simulink model "verify_Room_Floor_Heating_mdl"  (R2016b)
settings: Solver=ode15s  StartTime=0  StopTime=24*3600  MaxStep=900  RelTol=1e-3  EnableMultiTasking=on
libraries: carnot x8
settings Model: Creator=drhf  LastModifiedBy=drhf
settings DataIOCC: SaveFormat=Array  SignalLoggingSaveFormat=ModelDataLogs
settings OptimizationCC: ExpressionDepthLimit=2147483647  LifeSpan=inf
settings DebuggingCC: UnderspecifiedInitializationDetection=Classic  MergeDetectMultiDrivingBlocksExec=none  SolverPrmCheckMsg=warning  FcnCallInpInsideContextMsg=warning  StateNameClashWarn=warning  SFUnexpectedBacktrackingDiag=warning  SFNoUnconditionalDefaultTransitionDiag=warning  SFExecutionAtInitializationDiag=none
settings HardwareCC: ProdBitPerPointer=32  ProdBitPerSizeT=32  ProdBitPerPtrDiffT=32  ProdLargestAtomicFloat=None  ProdIntDivRoundTo=Undefined  ProdEndianess=Unspecified  ProdWordSize=32  ProdHWDeviceType=32-bit Generic
settings ModelReferenceCC: PropagateSignalLabelsOutOfModel=off
settings GRTTargetCC: TargetLangStandard=C89/C90 (ANSI)  GeneratePreprocessorConditionals=Disable all  CombineOutputUpdateFcns=off  GRTInterface=on
settings ConfigComp: CovMetricSettings=dw  CovHtmlReporting=on  CovSaveCumulativeToWorkspaceVar=on  CovSaveSingleToWorkspaceVar=on  CovExternalEMLEnable=off

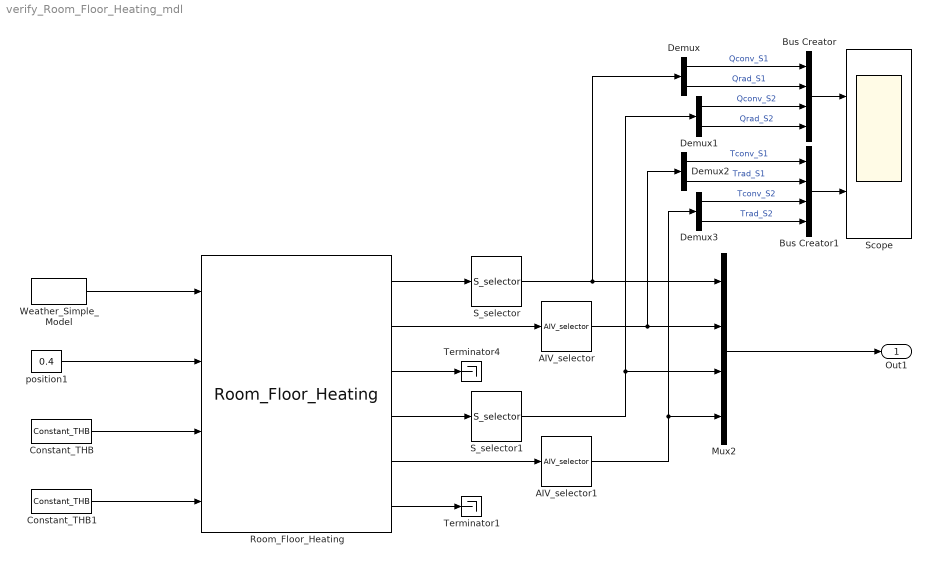
== system verify_Room_Floor_Heating_mdl ==
  AIV_selector : carnot/Outputs/AIV_selector  e1=off  e2=on  e3=on  e4=off  e5=off  e6=off  e7=off  e8=off  e9=off
  AIV_selector1 : carnot/Outputs/AIV_selector  e1=off  e2=on  e3=on  e4=off  e5=off  e6=off  e7=off  e8=off  e9=off
  Bus Creator : BusCreator  Inputs=4
  Bus Creator1 : BusCreator  Inputs=4
  Constant_THB : carnot/Source/Simple/Constant_THB  t=22  mdot=600/3600  p=1e5  mID=No Pressure Drop  fluid=Water  mix=0  mix2=0  mix3=0  dia=0.02  hgt=0
  Constant_THB1 : carnot/Source/Simple/Constant_THB  t=30  mdot=600/3600  p=1e5  mID=No Pressure Drop  fluid=Water  mix=0  mix2=0  mix3=0  dia=0.02  hgt=0
  Demux{,1..3} (4 alike) : Demux  Outputs=2
  Mux2 : Mux
  Room_Floor_Heating : carnot/Load/Houses/Room_Floor_Heating  t0=20  temp_neighbour=20
  S_selector : carnot/Outputs/S_selector  e1=off  e2=off  e3=off  e4=off  e5=off  e6=off  e7=on  e8=on  e9=off  e10=off  e11=off  e12=off  e13=off
  S_selector1 : carnot/Outputs/S_selector  e1=off  e2=off  e3=off  e4=off  e5=off  e6=off  e7=on  e8=on  e9=off  e10=off  e11=off  e12=off  e13=off
  Scope : Scope  NumInputPorts=2
  Terminator1 : Terminator
  Terminator4 : Terminator
  Weather_Simple_Model : carnot/Weather/Weather_Simple_Model  lat=60  Ibn=900  Idg=100  tamb=5  deltaTsky=-6  rh=50  precip="10e-3/24/3600           % 10 mm in 24 h"  cloud=0.125  p=1013e2  vw=1  wdir=270
  position1 : Constant  Value=0.4
  Out1 : Outport
  wires:
  Weather_Simple_Model/1 -> Room_Floor_Heating/1
  position1/1 -> Room_Floor_Heating/2
  Constant_THB1/1 -> Room_Floor_Heating/4
  Constant_THB/1 -> Room_Floor_Heating/3
  Room_Floor_Heating/3 -> Terminator4/1
  Room_Floor_Heating/6 -> Terminator1/1
  Room_Floor_Heating/1 -> S_selector/1
  Room_Floor_Heating/2 -> AIV_selector/1
  Room_Floor_Heating/4 -> S_selector1/1
  Room_Floor_Heating/5 -> AIV_selector1/1
  Bus Creator/1 -> Scope/1
  S_selector/1 -> Mux2/1, Demux/1
  S_selector1/1 -> Mux2/3, Demux1/1
  AIV_selector/1 -> Demux2/1, Mux2/2
  AIV_selector1/1 -> Mux2/4, Demux3/1
  Mux2/1 -> Out1/1
  Demux/1 -> Bus Creator/1  "Qconv_S1"
  Demux/2 -> Bus Creator/2  "Qrad_S1"
  Demux1/1 -> Bus Creator/3  "Qconv_S2"
  Demux1/2 -> Bus Creator/4  "Qrad_S2"
  Demux2/1 -> Bus Creator1/1  "Tconv_S1"
  Demux2/2 -> Bus Creator1/2  "Trad_S1"
  Demux3/2 -> Bus Creator1/4  "Trad_S2"
  Demux3/1 -> Bus Creator1/3  "Tconv_S2"
  Bus Creator1/1 -> Scope/2
